simulink model "MagLevNonLinearModel"  (R2015b)
settings: Solver=VariableStepAuto  StartTime=0.0  StopTime=10.0  RelTol=1e-3
values from neighbouring files (symbols this model uses):
  G = 9.81    [NonLinearSimulation.m]
  Km = 6.5308*10^-5    (= 6.5308e-05)    [NonLinearSimulation.m]
  L = 0.4125    [NonLinearSimulation.m]
  Mb = 0.068    [NonLinearSimulation.m]
  Rc = 10    [NonLinearSimulation.m]
  Rs = 1    [NonLinearSimulation.m]
undefined symbols (not defined in the file or in its folder): V
settings Model: Creator=Christopher  LastModifiedBy=Christopher
settings ConfigComp: CovModelRefEnable=Off

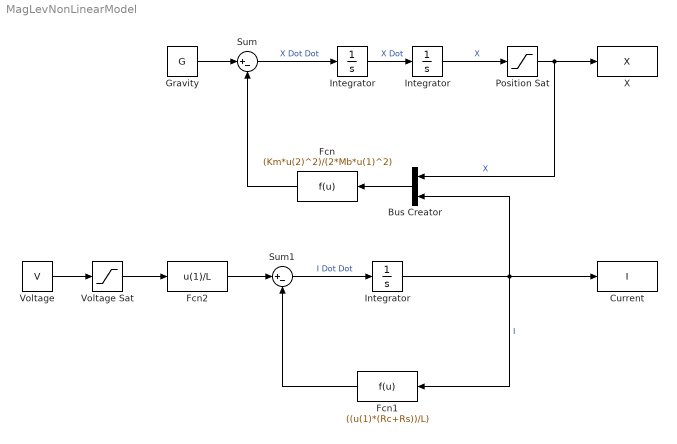
== system MagLevNonLinearModel ==
  Bus Creator : BusCreator  Inputs=2
  Current : ToWorkspace  VariableName=I  SaveFormat=Structure With Time  SampleTime=-1
  Fcn : Fcn  Expr=(Km*u(2)^2)/(2*Mb*u(1)^2)
  Fcn1 : Fcn  Expr=((u(1)*(Rc+Rs))/L)
  Fcn2 : Fcn  Expr=u(1)/L
  Gravity : Constant  Value=G
  Integrator : Integrator  InitialCondition=0.014
  "Integrator " : Integrator
  "Integrator " : Integrator
  Position Sat : Saturate  UpperLimit=0.014  LowerLimit=0.0000000000001
  Sum : Sum  Inputs=|+-
  Sum1 : Sum  Inputs=|+-
  Voltage : Constant  Value=V
  Voltage Sat : Saturate  UpperLimit=24  LowerLimit=-24
  X : ToWorkspace  VariableName=X  SaveFormat=Structure With Time  SampleTime=-1
  wires:
  Gravity/1 -> Sum/1
  Sum/1 -> "Integrator "/1  "X Dot Dot"
  "Integrator "/1 -> Integrator/1  "X Dot"
  Bus Creator/1 -> Fcn/1
  Fcn/1 -> Sum/2
  Integrator/1 -> Position Sat/1  "X"
  Position Sat/1 -> Bus Creator/1, X/1  "X"
  Fcn2/1 -> Sum1/1
  Sum1/1 -> "Integrator "/1  "I Dot Dot"
  Fcn1/1 -> Sum1/2
  "Integrator "/1 -> Bus Creator/2, Fcn1/1, Current/1  "I"
  Voltage/1 -> Voltage Sat/1
  Voltage Sat/1 -> Fcn2/1
